simulink model "vehiclemodel_public_0326"  (R2023b)
settings: Solver=FixedStepAuto  StartTime=0.0  StopTime=16  FixedStep=0.01  RelTol=1e-3
libraries: autolibshared x1
settings Model: Creator=StarY  LastModifiedBy=86182
settings OptimizationCC: DefaultParameterBehavior=Inlined  EnhancedBackFolding=on  PassReuseOutputArgsAs=Individual arguments  ZeroExternalMemoryAtStartup=off  ZeroInternalMemoryAtStartup=off  OptimizeBlockOrder=speed  DifferentSizesBufferReuse=on  OptimizationCustomize=off  EfficientTunableParamExpr=on
settings DebuggingCC: ParameterTunabilityLossMsg=error
settings HardwareCC: ProdBitPerLong=64  ProdHWDeviceType=Apple->ARM64  TargetBitPerPointer=64  TargetBitPerSizeT=64  TargetBitPerPtrDiffT=64  TargetLongLongMode=on  TargetIntDivRoundTo=Zero  TargetEndianess=LittleEndian  TargetWordSize=64  TargetHWDeviceType=MATLAB Host  ProdEqTarget=off
settings SFSimCC: MATLABDynamicMemAlloc=off
settings RTWCC: Description=Embedded Coder (host-based shared library target)  SystemTargetFile=ert_shrlib.tlc  TemplateMakefile=ert_default_tmf  GPUComputeCapability=5.0
settings CodeAppCC: ForceParamTrailComments=on  IgnoreCustomStorageClasses=off  OperatorAnnotations=on  SimulinkDataObjDesc=on  SFDataObjDesc=on  InsertBlockDesc=on
settings STFCustomTargetCC: MultiwordLength=256  GenerateSampleERTMain=on  ParMdlRefBuildCompliant=on  CompOptLevelCompliant=on  CombineOutputUpdateFcns=on  ERTCustomFileBanners=on  SupportNonInlinedSFcns=off  SupportVariableSizeSignals=on  MATLABClassNameForMDSCustomization=Simulink.SoftwareTarget.ERTCustomization  ModelStepFunctionPrototypeControlCompliant=on  UseToolchainInfoCompliant=on  SystemTargetFile=ert_shrlib.tlc
settings ERTTargetCC: TargetLangStandard=C99 (ISO)  GenerateSampleERTMain=on  ConcurrentExecutionCompliant=off  SupportContinuousTime=on  RemoveResetFunc=off  SupportVariableSizeSignals=on  CPPClassGenCompliant=off  InlinedParameterPlacement=NonHierarchical  RTWCAPISignals=on  RTWCAPIParams=on  RTWCAPIStates=on  RTWCAPIRootIO=on  ERTCustomFileTemplate=example_file_process.tlc

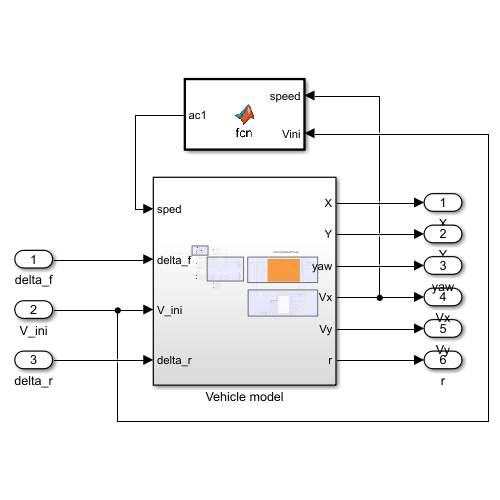
[thumbnail: Simulink's stored preview of the top-level diagram]
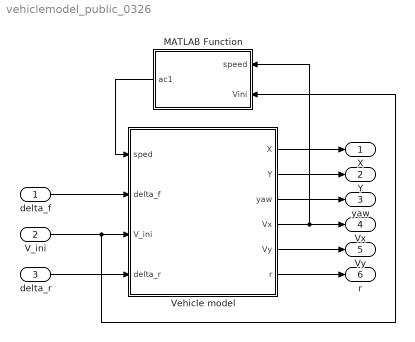
== system vehiclemodel_public_0326 ==
  delta_f : Inport
  V_ini : Inport  Port=2
  delta_r : Inport  Port=3
  MATLAB Function : MATLAB Function  TreatAsAtomicUnit=on
  Vehicle model : Subsystem
  X : Outport
  Y : Outport  Port=2
  yaw : Outport  Port=3
  Vx : Outport  Port=4
  Vy : Outport  Port=5
  r : Outport  Port=6
  wires:
  Vehicle model/6(r) -> r/1
  Vehicle model/1(X) -> X/1
  Vehicle model/3(yaw) -> yaw/1
  Vehicle model/2(Y) -> Y/1
  Vehicle model/5(Vy) -> Vy/1
  Vehicle model/4(Vx) -> Vx/1, MATLAB Function/1(speed)
  V_ini/1 -> Vehicle model/3(V_ini), MATLAB Function/2(Vini)
  delta_f/1 -> Vehicle model/2(delta_f)
  MATLAB Function/1(ac1) -> Vehicle model/1(sped)
  delta_r/1 -> Vehicle model/4(delta_r)

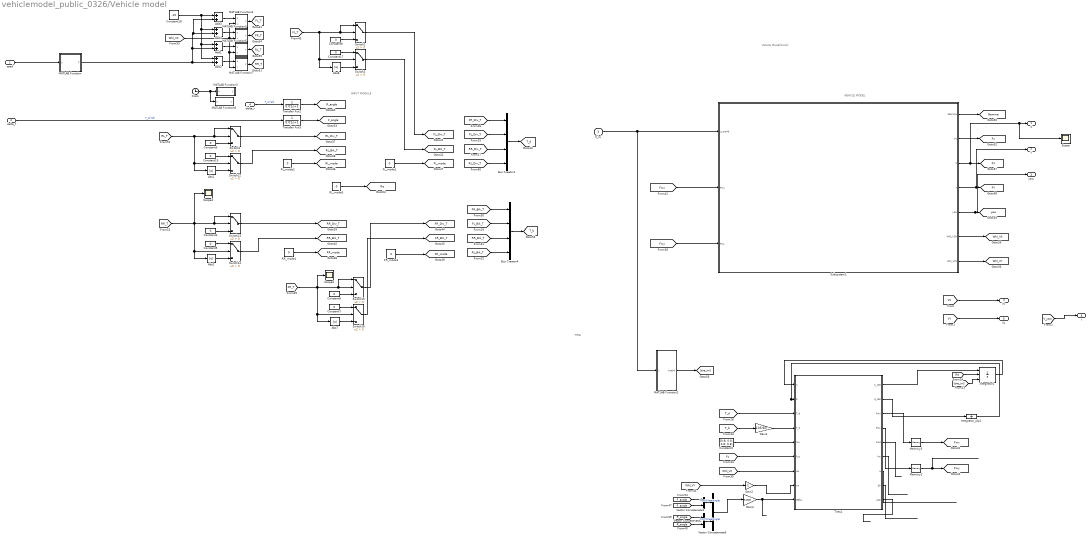
== system vehiclemodel_public_0326/Vehicle model ==
  note: INPUT MODULE
  note: TIRE
  note: VEHICLE MODEL
  note: Vehicle Model(Final)
  sped : Inport
  delta_f : Inport  Port=2
  V_ini : Inport  Port=3
  delta_r : Inport  Port=4
  Abs{1..2,7..8} (4 alike) : Abs  SaturateOnIntegerOverflow=off
  Add{1..4} (4 alike) : Sum
  Bus Creator1 : BusCreator  Inputs=4
  Bus Creator4 : BusCreator  Inputs=4
  Clock : Clock
  Constant{3..8,17,19} (8 alike) : Constant  Value=0
  Constant18 : Constant  Value=-15
  Constant2 : Constant  Value=[0.8; 0.8; 0.8; 0.8]
  FL_mode1 : Constant  Value=0
  FR_mode1 : Constant  Value=0
  Gain2 : Gain
  Gain3 : Gain  Gain=5.25/6
  Gain4 : Gain  Gain=105/60
  Integrator1 : Integrator  ExternalReset=rising  InitialConditionSource=external  LimitOutput=on  UpperSaturationLimit=[1e9;1e9;1e9;1e9;1e9;1e9]  LowerSaturationLimit=[-1e9;-1e9; -1e9;-1e9;-1e9;-1e9]
  Integrator_slip1 : Integrator  InitialCondition=zeros(8,1)  LimitOutput=on  UpperSaturationLimit=[1e9;1e9;1e9;1e9;1e9;1e9;1e9;1e9]  LowerSaturationLimit=[-1e9;-1e9;-1e9;-1e9;-1e9;-1e9;-1e9;-1e9]
  MATLAB Function : MATLAB Function  TreatAsAtomicUnit=on
  MATLAB Function2 : MATLAB Function  TreatAsAtomicUnit=on
  MATLAB Function3 : MATLAB Function  TreatAsAtomicUnit=on
  MATLAB Function4 : MATLAB Function  TreatAsAtomicUnit=on
  MATLAB Function5 : MATLAB Function  TreatAsAtomicUnit=on
  MATLAB Function6 : MATLAB Function  TreatAsAtomicUnit=on
  MATLAB Function7 : MATLAB Function  TreatAsAtomicUnit=on
  MATLAB Function8 : MATLAB Function  TreatAsAtomicUnit=on
  Memory2 : Memory
  Memory3 : Memory
  RL_mode2 : Constant  Value=0
  RL_mode3 : Constant  Value=0
  RR_mode1 : Constant  Value=0
  Scope : Scope
  Scope3 : Scope
  Scope4 : Scope
  Subsystem1 : Subsystem
  Switch{1..3,12..16} (8 alike) : Switch  Criteria=u2 > Threshold  SaturateOnIntegerOverflow=off  InputSameDT=off
  Tires1 : MATLAB Function  SystemSampleTime=0.001
  Transfer Fcn2 : TransferFcn  Denominator=[0.01 1]
  Transfer Fcn3 : TransferFcn  Denominator=[0.01 1]
  Vector Concatenate1 : Concatenate
  Vector Concatenate2 : Concatenate
  Vector Concatenate6 : Concatenate
  X : Outport
  Y : Outport  Port=2
  yaw : Outport  Port=3
  Vx : Outport  Port=4
  Vy : Outport  Port=5
  r : Outport  Port=6
  tag scope: FL_Brk_T=global, FL_Drv_T=global, FL_T=global, FL_mode=global, FR_Brk_T=global, FR_Drv_T=global, FR_T=global, FR_mode=global, F_angle=global, Fwx=global, Fwy=global, Fz=global, Gamma=global, PX=global, PY=global, RL_Brk_T=global, RL_Drv_T=global, RL_T=global, RL_mode=global, RR_Brk_T=global, RR_Drv_T=global, RR_T=global, RR_mode=global, R_angle=global, Re=global, T_b=global, T_d=global, Whl_VX=global, Whl_VY=global, yaw=global
  wires:
  Abs2/1 -> Switch14/3
  Memory3/1 -> [Fwx]
  Clock/1 -> MATLAB Function8/1(u), MATLAB Function3/1(u)
  FR_mode1/1 -> [FR_mode]
  [T_b] -> Gain4/1
  MATLAB Function4/1(y) -> [FL_T]
  Tires1/7(a) -> ?
  Constant18/1 -> Add2/1, Add1/1, Add4/1, Add3/1
  FL_mode1/1 -> [FL_mode]
  Add4/1 -> MATLAB Function5/1(u)
  Tires1/3(Fwx) -> Memory3/1
  Add3/1 -> MATLAB Function4/1(u)
  Gain3/1 -> Tires1/9(delta)
  MATLAB Function6/1(y) -> [RL_T]
  Add1/1 -> MATLAB Function6/1(u)
  [R_angle] -> Vector Concatenate2/1
  MATLAB Function/1(T) -> Add1/2, Add3/2, Add4/2, Add2/2
  MATLAB Function5/1(y) -> [FR_T]
  Add2/1 -> MATLAB Function7/1(u)
  Constant3/1 -> Switch3/3
  Constant2/1 -> Tires1/5(mu)
  Switch12/1 -> [RL_Brk_T]
  Vector Concatenate1/1 -> Vector Concatenate6/1  "FrontWheelAngles"
  Vector Concatenate2/1 -> Vector Concatenate6/2  "FrontWheelAngles"
  [R_angle] -> Vector Concatenate2/2
  Constant5/1 -> Switch14/1
  [Fz] -> Tires1/6(Fzs)
  Tires1/2(S_dot) -> Integrator_slip1/1
  V_ini/1 -> MATLAB Function2/1(v), Subsystem1/1(u_world)
  Tires1/5(kw0) -> ?
  Subsystem1/1(Gamma) -> [Gamma]
  Switch14/1 -> [RR_Brk_T]
  [RL_Drv_T] -> Bus Creator1/4
  [RL_T] -> Switch12/2, Abs1/1, Switch3/1, Switch3/2
  [RR_T] -> Scope3/1, Switch14/2, Abs2/1, Switch13/1, Switch13/2
  Abs7/1 -> Switch16/3
  Constant19/1 -> Switch12/1
  RL_mode2/1 -> [RL_mode]
  Gain4/1 -> Tires1/4(T_b)
  Constant7/1 -> Switch16/1
  Constant4/1 -> Switch13/3
  [FL_T] -> Switch2/2, Abs8/1, Switch1/1, Switch1/2
  [FL_Drv_T] -> Bus Creator1/2
  Constant8/1 -> Switch1/3
  Tires1/4(Fwy) -> Memory2/1
  [FR_Drv_T] -> Bus Creator1/1
  [RL_Brk_T] -> Bus Creator4/4
  [Whl_VY] -> Gain2/1
  Abs8/1 -> Switch2/3
  [tire_ini] -> Integrator1/3
  [Re] -> Integrator1/2
  [RR_Drv_T] -> Bus Creator1/3
  Bus Creator4/1 -> [T_b]
  [T_d] -> Tires1/3(T_d)
  Switch13/1 -> [RR_Drv_T]
  Memory2/1 -> [Fwy]
  [RR_Brk_T] -> Bus Creator4/3
  Integrator_slip1/1 -> Tires1/2(S)
  Constant6/1 -> Switch15/3
  [Whl_VX] -> Tires1/7(uw)
  Switch1/1 -> [FL_Drv_T]
  [FR_Brk_T] -> Bus Creator4/1
  Transfer Fcn2/1 -> [R_angle]
  Constant17/1 -> Switch2/1
  Switch2/1 -> [FL_Brk_T]
  Switch16/1 -> [FR_Brk_T]
  Vector Concatenate6/1 -> Gain3/1
  Bus Creator1/1 -> [T_d]
  Switch3/1 -> [RL_Drv_T]
  [Fwx] -> Subsystem1/2(Fwx)
  MATLAB Function7/1(y) -> [RR_T]
  Integrator1/1 -> Tires1/1(X)
  RR_mode1/1 -> [RR_mode]
  Tires1/6(kw) -> ?
  [F_angle] -> Vector Concatenate1/1
  [Fwy] -> Subsystem1/3(Fwy)
  Abs1/1 -> Switch12/3
  Transfer Fcn3/1 -> [F_angle]
  Tires1/8(a0) -> ?
  [FR_T] -> Switch16/2, Abs7/1, Scope4/1, Switch15/1, Switch15/2
  [F_angle] -> Vector Concatenate1/2
  [FL_Brk_T] -> Bus Creator4/2
  Subsystem1/7(Whl_V0Y) -> [Whl_VY]
  Subsystem1/6(Whl_V0X) -> [Whl_VX]
  Subsystem1/5(yaw) -> yaw/1, [yaw]
  RL_mode3/1 -> [Re]
  MATLAB Function2/1(tireini) -> [tire_ini]
  Tires1/1(X_dot) -> Integrator1/1
  Switch15/1 -> [FR_Drv_T]
  Tires1/9(a10) -> ?
  Subsystem1/2(Fz) -> [Fz]
  Gain2/1 -> Tires1/8(vw)
  [Whl_VX] -> MATLAB Function7/2(v), MATLAB Function6/2(v), MATLAB Function5/2(v), MATLAB Function4/2(v)
  Subsystem1/3(X) -> Scope/1, X/1, [PX]
  sped/1 -> MATLAB Function/1(u)
  delta_f/1 -> Transfer Fcn3/1  "F_a(rad)"
  Subsystem1/4(Y) -> Y/1, [PY]
  [VX] -> Vx/1
  [VY] -> Vy/1
  [V_yaw] -> r/1
  delta_r/1 -> Transfer Fcn2/1  "F_a(rad)"

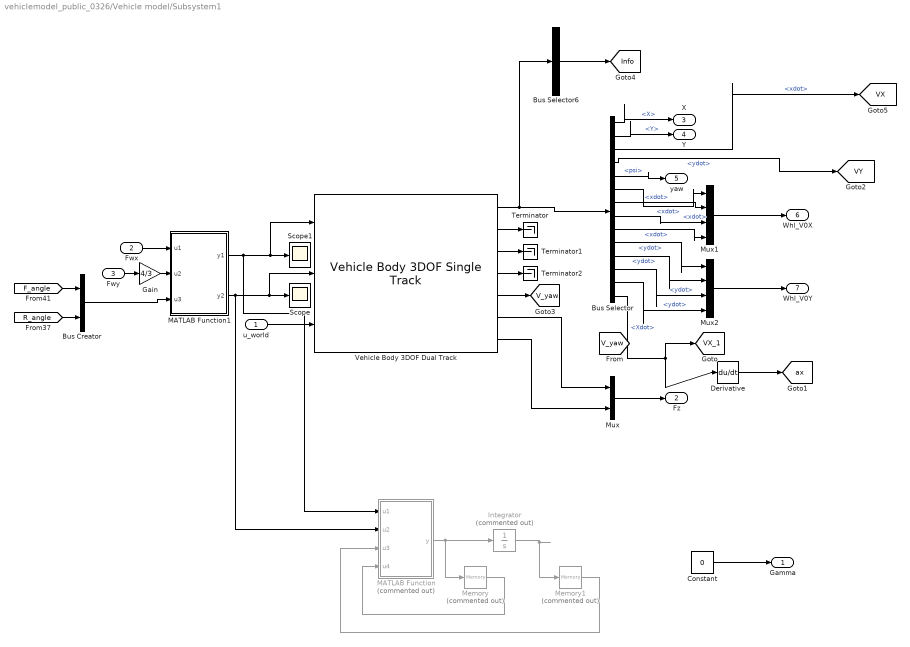
== system vehiclemodel_public_0326/Vehicle model/Subsystem1 ==
  u_world : Inport
  Fwx : Inport  Port=2
  Fwy : Inport  Port=3
  Bus Creator : BusCreator  Inputs=2
  Bus Selector : BusSelector  OutputSignals=InertFrm.Geom.Disp.X,InertFrm.Geom.Disp.Y,BdyFrm.Cg.Vel.xdot,BdyFrm.Cg.Vel.ydot,InertFrm.Cg.Ang.psi,BdyFrm.FrntAxl.Lft.Vel.xdot,BdyFrm.FrntAxl.Rght.Vel.xdot,BdyFrm.RearAxl.Lft.Vel.xdot,BdyFrm.RearAxl.Rght.Vel.xdot,BdyFrm.FrntAxl.Lft.Vel.ydot,BdyFrm.FrntAxl.Rght.Vel.ydot,BdyFrm.RearAxl.Lft.Vel.ydot,BdyFrm.RearAxl.Rght.Vel.ydot,InertFrm.Geom.Vel.Xdot
  Bus Selector6 : BusSelector  OutputSignals=InertFrm.Geom.Disp.X,InertFrm.Geom.Disp.Y,BdyFrm.Cg.Vel.xdot,BdyFrm.Cg.Vel.ydot,InertFrm.Cg.Ang.psi,BdyFrm.Cg.AngVel.r  OutputAsBus=on
  Constant : Constant  Value=0
  Derivative : Derivative
  Gain : Gain  Gain=4/3
  Integrator : Integrator  Commented=on  LimitOutput=on  UpperSaturationLimit=pi  LowerSaturationLimit=-pi
  MATLAB Function : MATLAB Function  Commented=on  TreatAsAtomicUnit=on
  MATLAB Function1 : MATLAB Function  TreatAsAtomicUnit=on
  Memory : Memory  Commented=on
  Memory1 : Memory  Commented=on
  Mux : Mux  Inputs=2
  Mux1 : Mux
  Mux2 : Mux
  Scope : Scope
  Scope1 : Scope
  Terminator : Terminator
  Terminator1 : Terminator
  Terminator2 : Terminator
  Vehicle Body 3DOF Dual Track : autolibshared/Vehicle Body 3DOF Single Track  trackMode=Dual  inputMode=External forces  frontSteerMode=off  rearSteerMode=off  windMode=off  muMode=off  extFMode=off  extMMode=off  htchFMode=off  htchMMode=off  extXo=off  extpsio=off  extxdoto=on  extro=off  extYo=off  extTamb=off  extydoto=off  aMode=2  NF=2  NR=2  m=1350  a=1.4  b=1.6  h=0.35  dh=1  hh=0.2  X_o=0.11  xdot_o=80/3.6  CalphaMode=off  sigmaMode=on  d=0  hl=0  w=[1.4,1.4]  Cy_f=12e3  Cy_r=11e3  sigma_f=.1  sigma_r=.1  alpha_f_brk=[-.1 .1]  Cy_f_data=[-9e3 9e3]  alpha_r_brk=[-.1 .1]  Cy_r_data=[-9e3 9e3]  Y_o=0  ydot_o=0  Izz=1536  psi_o=0  r_o=0  Af=2  Cd=.3  Cl=.1  Cpm=.1  beta_w=[0 0.01:0.01:0.3]  Cs=[0:0.03:0.9]  Cym=[0 1e-6:0.01:0.3]  Pabs=101325  Tair=273  g=9.81  mu=1  xdot_tol=.01  Fznom=5000  Fxtire_sat=7e4  Fytire_sat=7e4  longOff=0  latOff=0  vertOff=0  wrapAng=off
  Gamma : Outport
  Fz : Outport  Port=2
  X : Outport  Port=3
  Y : Outport  Port=4
  yaw : Outport  Port=5
  Whl_V0X : Outport  Port=6
  Whl_V0Y : Outport  Port=7
  tag scope: Info=global, VX=global, VX_1=global, VY=global, V_yaw=global, ax=global
  wires:
  Bus Selector/2 -> Y/1  "<Y>"
  Vehicle Body 3DOF Dual Track/7 -> Mux/2
  Vehicle Body 3DOF Dual Track/6 -> Mux/1
  Mux/1 -> Fz/1
  Fwx/1 -> MATLAB Function1/1(u1)
  Fwy/1 -> Gain/1
  MATLAB Function1/2(y2) -> MATLAB Function/2(u2), Vehicle Body 3DOF Dual Track/2, Scope/1
  u_world/1 -> Vehicle Body 3DOF Dual Track/3
  Bus Selector/4 -> [VY]  "<ydot>"
  Bus Selector/3 -> [VX]  "<xdot>"
  Bus Selector/1 -> X/1  "<X>"
  Bus Selector/5 -> yaw/1  "<psi>"
  Integrator/1 -> Memory1/1
  Bus Selector/6 -> Mux1/1  "<xdot>"
  Bus Selector/7 -> Mux1/2  "<xdot>"
  Bus Selector/8 -> Mux1/3  "<xdot>"
  Bus Selector/9 -> Mux1/4  "<xdot>"
  Mux1/1 -> Whl_V0X/1
  Bus Selector/10 -> Mux2/1  "<ydot>"
  Bus Selector/11 -> Mux2/2  "<ydot>"
  Mux2/1 -> Whl_V0Y/1
  Bus Selector/13 -> Mux2/4  "<ydot>"
  Bus Selector/12 -> Mux2/3  "<ydot>"
  MATLAB Function1/1(y1) -> Scope1/1, Vehicle Body 3DOF Dual Track/1, MATLAB Function/1(u1)
  Vehicle Body 3DOF Dual Track/5 -> [V_yaw]
  [F_angle] -> Bus Creator/1
  [R_angle] -> Bus Creator/2
  Bus Creator/1 -> MATLAB Function1/3(u3)
  Vehicle Body 3DOF Dual Track/2 -> Terminator/1
  Vehicle Body 3DOF Dual Track/3 -> Terminator1/1
  Vehicle Body 3DOF Dual Track/4 -> Terminator2/1
  MATLAB Function/1(y) -> Memory/1, Integrator/1
  Memory/1 -> MATLAB Function/4(u4)
  Memory1/1 -> MATLAB Function/3(u3)
  Constant/1 -> Gamma/1
  Gain/1 -> MATLAB Function1/2(u2)
  Bus Selector/14 -> Derivative/1, [VX_1]  "<Xdot>"
  Derivative/1 -> [ax]
  Vehicle Body 3DOF Dual Track/1 -> Bus Selector6/1, Bus Selector/1
  Bus Selector6/1 -> [Info]

== matlab function vehiclemodel_public_0326/Vehicle model/Subsystem1/MATLAB Function ==
  data: u1 input; y output; u2 input; u3 input; u4 input
function y = fcn(u1,u2,u3,u4)
Fy_sum = u1(2) + u1(4) + u2(2) + u2(4);
Mx = 1270*9.8*0.31*u3 + (-5000*u4-44000*u3) + (-5000*u4-44000*u3);
y = (-Fy_sum*1270*0.31 + 1300*Mx)/(1300*(440.6+1850*0.48^2)-1270^2*0.31^2);

== matlab function vehiclemodel_public_0326/Vehicle model/Subsystem1/MATLAB Function1 ==
  data: u1 input; y1 output; u2 input; y2 output; u3 input
function [y1,y2] = fcn(u1,u2,u3)
delta1 = u3(1); delta2 = u3(2);
kFx = 1;
kFy = 1;
Fx1 = (cos(delta1)*u1(1)*kFx-sin(delta1)*u2(1)*kFy);
Fy1 = (sin(delta1)*u1(1)*kFx+cos(delta1)*u2(1)*kFy);
Fx2 = (cos(delta1)*u1(2)*kFx-sin(delta1)*u2(2)*kFy);
Fy2 = (sin(delta1)*u1(2)*kFx+cos(delta1)*u2(2)*kFy);
y1 = [Fx1,Fy1;Fx2,Fy2];
Fx3 = (cos(delta2)*u1(3)*kFx-sin(delta2)*u2(3)*kFy);
Fy3 = (sin(delta2)*u1(3)*kFx+cos(delta2)*u2(3)*kFy);
Fx4 = (cos(delta2)*u1(4)*kFx-sin(delta2)*u2(4)*kFy);
Fy4 = (sin(delta2)*u1(4)*kFx+cos(delta2)*u2(4)*kFy);
y2 = [Fx3,Fy3;Fx4,Fy4];

== matlab function vehiclemodel_public_0326/Vehicle model/Tires1 ==
  data: X input size=6; S input; T_d input double size=4; T_b input; mu input double size=4; Fzs input; X_dot output double size=6; S_dot output; uw input size=4; vw input size=4; Fwx output double size=4; Fwy output double size=4; delta input size=4; kw0 output; kw output; a output; a0 output; a10 output
% 轮胎模型（carsim_215_55_r17）
% V0.0.3 20211001 xiataokai 修改回正力跳变问题
% V0.0.4 20211008 xiataokai 加入更多状态维度

function [X_dot, S_dot, Fwx, Fwy , kw0, kw, a,a0,a10]    = tir(X, S, T_d, T_b, mu, Fzs, uw, vw, delta)
a=0
a10 = -(atan(vw(2)/abs(uw(2))));
% delta的单位是rad
% Effective roling radius, m
Rw = 0.325; 
% Tire inertial, kg*m^2
Iw = 1.5; 
% Tire camber angle, deg
gamma0 = 0;
% Tire Rolling Resistance1, -
Rr_c = 0.0038; 
% Tire Rolling Resistance2, s/m
Rr_v = 0.000026/3.6; 
% Minimum tire logitudinal speed for slip calculation CTM(29), m/s 
Vmin = 0.5/3.6; 
% Relaxation length for lateral slip, m
Ly = 0.5; 
% Relaxation length for logitudinal slip, m
Lx = 0.5; 

% Differential shaft to left wheel intertial, kg-m2
Diff_IL = 0.009;
% Differential shaft to right wheel intertial, kg-m2
Diff_IR = 0.009;


% Slip rate and slip angle
k1 = Rw*X(1)/max(abs(uw(1)),Vmin)-1;
k2 = Rw*X(2)/max(abs(uw(2)),Vmin)-1;
k3 = Rw*X(3)/max(abs(uw(3)),Vmin)-1;
k4 = Rw*X(4)/max(abs(uw(4)),Vmin)-1;

if vw(1) >= 0
    a1 = -(atan(vw(1)/max(abs(uw(1)),Vmin)) - delta(1));  % 20210809符号问题，这里的轮胎侧偏角取负才是对的  
else
    a1 = -(atan(vw(1)/max(abs(uw(1)),Vmin)) - delta(1)); %+ sign(vw(1))*pi; 
end
if vw(2) >= 0
    a2 = -(atan(vw(2)/max(abs(uw(2)),Vmin)) - delta(2));  % 20210809符号问题，这里的轮胎侧偏角取负才是对的  
else
    a2 = -(atan(vw(2)/max(abs(uw(2)),Vmin)) - delta(2)); %+ sign(vw(2))*pi; 
end
if vw(3) >= 0
    a3 = -(atan(vw(3)/max(abs(uw(3)),Vmin)) - delta(3));  % 20210809符号问题，这里的轮胎侧偏角取负才是对的  
else
    a3 = -(atan(vw(3)/max(abs(uw(3)),Vmin)) - delta(3)); %+ sign(vw(3))*pi; 
end
if vw(4) >= 0
    a4 = -(atan(vw(4)/max(abs(uw(4)),Vmin)) - delta(4));  % 20210809符号问题，这里的轮胎侧偏角取负才是对的  
else
    a4 = -(atan(vw(4)/max(abs(uw(4)),Vmin)) - delta(4)); %+ sign(vw(4))*pi; 
end

if a1 >= pi/2
    a1 = pi - a1;
elseif a1 <= -pi/2
    a1 = -pi -a1;
else
    a1 = a1;
end
if a2 >= pi/2
    a2 = pi - a2;
elseif a1 <= -pi/2
    a2 = -pi -a2;
else
    a2 = a2;
end
if a3 >= pi/2
    a3 = pi - a3;
elseif a3 <= -pi/2
    a3 = -pi -a3;
else
    a3 = a3;
end
if a4 >= pi/2
    a4 = pi - a4;
elseif a4 <= -pi/2
    a4 = -pi -a4;
else
    a4 = a4;
end

a0 = [a1,a2,a3,a4];

kw0 = zeros(4,1); kw0(1) = k1; kw0(2) = k2; kw0(3)= k3; kw0(4) = k4;

% Lagged slip rate and slip angle (Tire transients)
S_dot = zeros(8,1);
S_dot(1) = max(abs(uw(1)),Vmin)/Lx*(k1-S(1)); % CTM(28)
S_dot(2) = max(abs(uw(2)),Vmin)/Lx*(k2-S(2));
S_dot(3) = max(abs(uw(3)),Vmin)/Lx*(k3-S(3));
S_dot(4) = max(abs(uw(4)),Vmin)/Lx*(k4-S(4));
% S_dot(5) = max(abs(uw(1)),Vmin)/Ly*(tan(a1)-S(5)); % CTM(27)
% S_dot(6) = max(abs(uw(2)),Vmin)/Ly*(tan(a2)-S(6));
% S_dot(7) = max(abs(uw(3)),Vmin)/Ly*(tan(a3)-S(7));
% S_dot(8) = max(abs(uw(4)),Vmin)/Ly*(tan(a4)-S(8));
% a = [atan(S(5)),atan(S(6)),atan(S(7)),atan(S(8))];
kw = zeros(4,1); kw(1) = k1; kw(2) = k2; kw(3)= k3; kw(4) = k4;
% Lateral force, longitudinal force, aligning torque
Fwx = zeros(4,1); Fwy = zeros(4,1); %Mwz = zeros(4,1); 
% [Fwx(1), Fwy(1)] = Tire(Fzs(1), S(1), atan(S(5)), mu(1), + gamma0);
% [Fwx(2), Fwy(2)] = Tire(Fzs(2), S(2), atan(S(6)), mu(2), - gamma0);
% [Fwx(3), Fwy(3)] = Tire(Fzs(3), S(3), atan(S(7)), mu(3), gamma0);
% [Fwx(4), Fwy(4)] = Tire(Fzs(4), S(4), atan(S(8)), mu(4), -gamma0);
[Fwx(1), Fwy(1)] = Tire(Fzs(1), S(1), a1, mu(1), + gamma0);
[Fwx(2), Fwy(2)] = Tire(Fzs(2), S(2), a2, mu(2), - gamma0);
[Fwx(3), Fwy(3)] = Tire(Fzs(3), S(3), a3, mu(3), gamma0);
[Fwx(4), Fwy(4)] = Tire(Fzs(4), S(4), a4, mu(4), -gamma0);
% Tire dynamics
X_dot = zeros(6,1);
I_drv = 5;
M_LF = (-T_b(1)-Rw*Fwx(1)-0*Fzs(1)*Rw*(Rr_c+Rr_v*uw(1)));
M_RF = (-T_b(2)-Rw*Fwx(2)-0*Fzs(2)*Rw*(Rr_c+Rr_v*uw(2)));
X_dot(1) = (T_d(1) + M_LF + I_drv*(M_LF-M_RF)/(Iw+Diff_IL))/(Iw+Diff_IL+I_drv*(1+(Iw+Diff_IL)/(Iw+Diff_IR)));
X_dot(2) = (T_d(2) + M_RF + I_drv*(M_RF-M_LF)/(Iw+Diff_IL))/(Iw+Diff_IR+I_drv*(1+(Iw+Diff_IR)/(Iw+Diff_IL)));
X_dot(3) = (T_d(3)-T_b(3)-Rw*Fwx(3)-0*Fzs(3)*Rw*(Rr_c+Rr_v*uw(3)))/Iw;
X_dot(4) = (T_d(4)-T_b(4)-Rw*Fwx(4)-0*Fzs(4)*Rw*(Rr_c+Rr_v*uw(4)))/Iw;
X_dot(5) = X(1);
X_dot(6) = X(2);


1;
end

function [Fx, Fy] = Tire(Fz, k, a, mu, gamma)
% Magical formular model of the tires，fitted from CarSim 215/55 R17
% Fz(N) vertical load 
% k(0~1) slip rate
% a(deg) slip angle
% mu(0~1) friction coeeficient
% gamma(deg) camber angle
a = a/pi*180;
mu0 = 1;
Fz0 = 4.7807e+03;
PFxB0 = 22.1951;
PFxC0 = 1.3997;
PFxD0 = 4.6565e+03;
PFxE0 = 0.5490;
PFyB0 = 0.1390;
PFyC0 = 2.2067;
PFyD0 = 4.6603e+03;
PFyE0 = 1.0047;
PMzB0 = 0.2665;
PMzC0 = 2.1415;
PMzD0 = 72.4154;
PMzE0 = -6.9391;
PCFkappa0 = 15.3932*6.6204*Fz0*sin(2*atan(Fz0/6.6204/Fz0));
PCFalpha0 = 0.1535*5.5010*Fz0*sin(2*atan(Fz0/5.5010/Fz0));
PCMalpha0 = (0.0290*(Fz0/Fz0).^0.0530).*PCFalpha0;
PCFkappa = 15.3932*6.6204*Fz0*sin(2*atan(Fz/6.6204/Fz0));
PCFalpha = 0.1535*5.5010*Fz0*sin(2*atan(Fz/5.5010/Fz0));
%PCMalpha = (0.0290*(Fz/Fz0).^0.0530).*PCFalpha;
PCMalpha = PCFalpha;
PCFgamma = 0.010*Fz;
PCMgamma = 0.10*(0.07)^2/0.3*PCFkappa;  % 系数取值具体多少有待商榷，书上Table4.1给的0.3，这里改成0.10
% 横纵向联合全滑移
astar = a+PCFgamma/PCFalpha*gamma; %4.29
sx = k/(1.0+k+1e-7);
systar = tan(astar/180*pi)/(1.0+k+1e-7);
sstar = sqrt(sx^2+systar^2)+1e-7;
sxeq = sstar*sign(sx);
syeq = sstar*sign(systar);   % 这个sign参考了CarSim Tire_Models.pdf P34**
keq = sxeq/(1-sxeq+1e-7)*(PCFkappa/PCFkappa0)*(mu0/mu)*(Fz0/Fz);  % 这个式子用4.30还是4.30a有待考虑，这是4.30
aeq = atan(syeq)/pi*180*(PCFalpha/PCFalpha0)*(mu0/mu)*(Fz0/Fz);
% 横向力、纵向力、回正力计算
Fx = abs(sx/sstar)*(mu/mu0)*(Fz/Fz0)...
    *PFxD0*sin(PFxC0*atan(PFxB0*keq-PFxE0*(PFxB0*keq-atan(PFxB0*keq))));
Fy = abs(systar/sstar)*(mu/mu0)*(Fz/Fz0)...  % 这个abs与**的sign配套，不然Fx,Fy计算的符号不对了
    *PFyD0*sin(PFyC0*atan(PFyB0*aeq-PFyE0*(PFyB0*aeq-atan(PFyB0*aeq))))*sign(k+1);
Mzr = (PCMgamma+PCFgamma*PCMalpha/PCFalpha)./(1+100*(syeq).^2)*gamma/180*pi;  % 系数取值具体多少有待商榷
Mzcouple = -0.3*0.08*Fx*Fy/Fz0 - 0*0.08*Fx - 4*0.07*Fx*gamma/180*pi;  % 系数取值具体多少有待商榷
Mz = -abs(systar/sstar)*(mu/mu0)*(Fz/Fz0)*(PCMalpha/PCMalpha0)*(PCFalpha0/PCFalpha)...
    *PMzD0*sin(PMzC0*atan(PMzB0*aeq-PMzE0*(PMzB0*aeq-atan(PMzB0*aeq))))...
    +Mzr+Mzcouple;
1;
end

== matlab function vehiclemodel_public_0326/MATLAB Function ==
  data: speed input; ac1 output; Vini input
function ac1 = fcn(speed,Vini)

ac1 = 0.2*(Vini+0.35 - speed);

if ac1 > 0
    ac = ac1;
    dc = 0;
else
    dc = abs(ac1);
    ac = 0
end

== matlab function vehiclemodel_public_0326/Vehicle model/MATLAB Function2 ==
  data: v input; tireini output
function tireini = fcn(v)
R = 0.325;
w = v/R;
tireini = [w; w; w; w; 0; 0];
end

== matlab function vehiclemodel_public_0326/Vehicle model/MATLAB Function3 ==
  data: u input; y output
function y = fcn(u)
% if u <= 0.3+0.1
%     y = 5/180*pi;
% elseif u <=0.65+0.1
%     y = -20/180*pi;
% elseif u <=0.82+0.1
%     y = 0;
% elseif u <=1.5+0.1
%     y = 10/180*pi;
% 
% else
%     y = 0;
% end
 y =10/180*pi;

== matlab function vehiclemodel_public_0326/Vehicle model/MATLAB Function4 ==
  data: u input; y output; v input
function y = fcn(u,v)
if v(2) >= 0
    y = u;
else
    y = -u;
end

== matlab function vehiclemodel_public_0326/Vehicle model/MATLAB Function5 ==
  data: u input; y output; v input
function y = fcn(u,v)
if v(1) >= 0
    y = u;
else
    y = -u;
end

== matlab function vehiclemodel_public_0326/Vehicle model/MATLAB Function6 ==
  data: u input; y output; v input
function y = fcn(u,v)
if v(4) >= 0
    y = u;
else
    y = -u;
end

== matlab function vehiclemodel_public_0326/Vehicle model/MATLAB Function ==
  data: u input; T output
function T = fcn(u)
if u >=0
    T = u*500;
else
    T = u*600;
end

== matlab function vehiclemodel_public_0326/Vehicle model/MATLAB Function7 ==
  data: u input; y output; v input
function y = fcn(u,v)
if v(3) >= 0
    y = u;
else
    y = -u;
end

== matlab function vehiclemodel_public_0326/Vehicle model/MATLAB Function8 ==
  data: u input; y output
function y = fcn(u)
if u <= 0.3+0.1
    y = 0;
elseif u <=0.65+0.1
    y = 20/180*pi;
elseif u <=0.82+0.1
    y = 0;
elseif u <=1.5+0.1
    y = -10/180*pi;

else
    y = 0;
end
